simulink model "ON"  (R2025b)
settings: Solver=VariableStepAuto  StartTime=0.0  StopTime=300  FixedStep=0.5  RelTol=1e-3
InitFcn:
  | mdlWks = get_param(gcs,'ModelWorkspace');
  | a = getVariable(mdlWks,'a');
  | b = getVariable(mdlWks,'b');
  | c = getVariable(mdlWks,'c');
StopFcn:
  | fTraj = findobj("Tag","asbAUVTrajectory");
  | 
  | if isempty(fTraj)
  |    fTraj = figure("Tag","asbAUVTrajectory");
  |    axes(fTraj);
  | end
  | 
  | axTraj= gca(fTraj);
  | 
  | if exist('PositionData', 'var')
  |    plot3(axTraj,PositionData(1,1),PositionData(1,2),PositionData(1,3),'r*')
  |    hold on
  |    plot3(axTraj,PositionData(:,1),PositionData(:,2),PositionData(:,3));
  |    plot3(axTraj,PositionData(end,1),PositionData(end,2),PositionData(end,3),'g*');
  | 
  |    axTraj.XLim = [0 15];
  |    axTraj.YLim = [-10 2];
  |    axTraj.ZLim = [-2 12];
  |    axTraj.XLabel.String = 'X (m)';
  |    axTraj.YLabel.String = 'Y (m)';
  |    axTraj.ZLabel.String = 'Z (m)';
  |    grid on
  |    hold off
  | 
  |    legend(axTraj,{'Start Point','Trajectory','End Point'});
  | end
model workspace (MAT data in the model file):
  a = 1
  b = 0
  c = 1
libraries: asbAUVlib x28, dspfdesign x6, slpidlib x6, aerolibobsolete x1, aerolibasang x1, sharedutil x1, aerolibnav x1, SignalEditorBlockLib x1
(part 3 of 3)

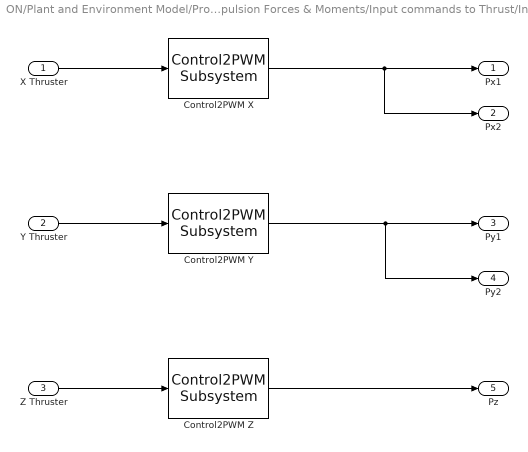
== system ON/Plant and Environment Model/Propulsion Forces & Moments/Input commands to Thrust/Input Commands to PWM ==
  X Thruster : Inport
  Y Thruster : Inport  Port=2
  Z Thruster : Inport  Port=3
  Control2PWM X : asbAUVlib/Control2PWM Subsystem  SystemSampleTime=-1  VariantActivationTime=update diagram  EmptyChoice=off  PassThrough=off  PassThroughVariantControl=(default)  EmptyChoiceVariantControl=(default)  AllowFlexibleInterface=on  Latency=0  AutoFrameSizeCalculation=off
  Control2PWM Y : asbAUVlib/Control2PWM Subsystem  SystemSampleTime=-1  VariantActivationTime=update diagram  EmptyChoice=off  PassThrough=off  PassThroughVariantControl=(default)  EmptyChoiceVariantControl=(default)  AllowFlexibleInterface=on  Latency=0  AutoFrameSizeCalculation=off
  Control2PWM Z : asbAUVlib/Control2PWM Subsystem  SystemSampleTime=-1  VariantActivationTime=update diagram  EmptyChoice=off  PassThrough=off  PassThroughVariantControl=(default)  EmptyChoiceVariantControl=(default)  AllowFlexibleInterface=on  Latency=0  AutoFrameSizeCalculation=off
  Px1 : Outport  VectorParamsAs1DForOutWhenUnconnected=off
  Px2 : Outport  Port=2  VectorParamsAs1DForOutWhenUnconnected=off
  Py1 : Outport  Port=3  VectorParamsAs1DForOutWhenUnconnected=off
  Py2 : Outport  Port=4  VectorParamsAs1DForOutWhenUnconnected=off
  Pz : Outport  Port=5  VectorParamsAs1DForOutWhenUnconnected=off
  wires:
  Control2PWM Z/1 -> Pz/1
  Y Thruster/1 -> Control2PWM Y/1
  Control2PWM Y/1 -> Py1/1, Py2/1
  Z Thruster/1 -> Control2PWM Z/1
  Control2PWM X/1 -> Px1/1, Px2/1
  X Thruster/1 -> Control2PWM X/1

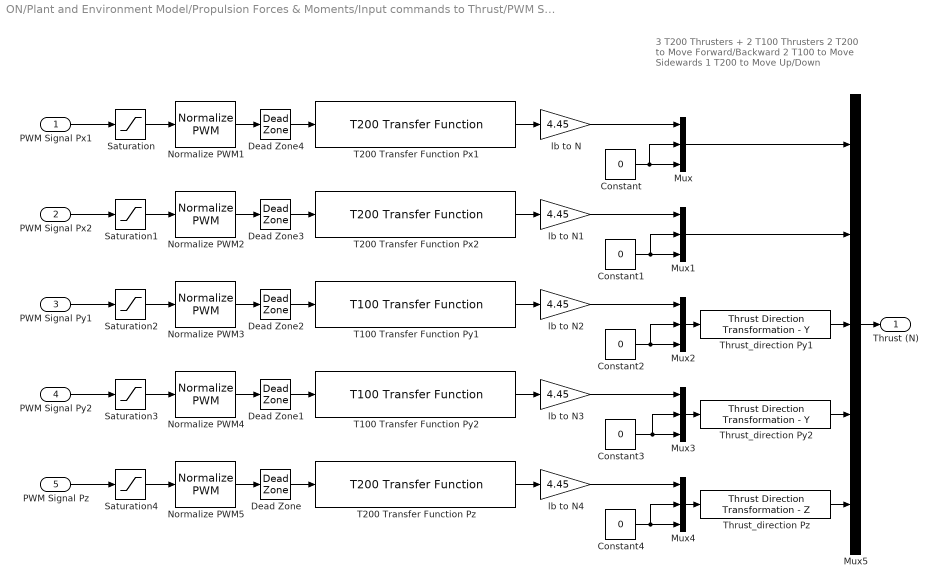
== system ON/Plant and Environment Model/Propulsion Forces & Moments/Input commands to Thrust/PWM Signals to Thrust  ==
  note: 3 T200 Thrusters + 2 T100 Thrusters
      |
      | 2 T200 to Move Forward/Backward
      | 2 T100 to Move Sidewards
      | 1 T200 to Move Up/Down
  PWM Signal Px1 : Inport
  PWM Signal Px2 : Inport  Port=2
  PWM Signal Py1 : Inport  Port=3
  PWM Signal Py2 : Inport  Port=4
  PWM Signal Pz : Inport  Port=5
  Constant{,1..4} (5 alike) : Constant  Value=0
  Dead Zone{,2..4} (4 alike) : DeadZone  LowerValue=-10  UpperValue=+10
  Dead Zone1 : DeadZone  LowerValue=-10  UpperValue=10
  Mux{,1..4} (5 alike) : Mux  Inputs=3
  Mux5 : Mux  Inputs=5
  Normalize PWM{1..5} (5 alike) : asbAUVlib/Normalize PWM  SystemSampleTime=-1  VariantActivationTime=update diagram  EmptyChoice=off  PassThrough=off  PassThroughVariantControl=(default)  EmptyChoiceVariantControl=(default)  AllowFlexibleInterface=on  Latency=0  AutoFrameSizeCalculation=off
  Saturation{,1..4} (5 alike) : Saturate  UpperLimit=1900  LowerLimit=1100
  T100 Transfer Function Py1 : asbAUVlib/T100 Transfer Function  SystemSampleTime=-1  VariantActivationTime=update diagram  EmptyChoice=off  PassThrough=off  PassThroughVariantControl=(default)  EmptyChoiceVariantControl=(default)  AllowFlexibleInterface=on  Latency=0  AutoFrameSizeCalculation=off
  T100 Transfer Function Py2 : asbAUVlib/T100 Transfer Function  SystemSampleTime=-1  VariantActivationTime=update diagram  EmptyChoice=off  PassThrough=off  PassThroughVariantControl=(default)  EmptyChoiceVariantControl=(default)  AllowFlexibleInterface=on  Latency=0  AutoFrameSizeCalculation=off
  T200 Transfer Function Px1 : asbAUVlib/T200 Transfer Function  SystemSampleTime=-1  VariantActivationTime=update diagram  EmptyChoice=off  PassThrough=off  PassThroughVariantControl=(default)  EmptyChoiceVariantControl=(default)  AllowFlexibleInterface=on  Latency=0  AutoFrameSizeCalculation=off
  T200 Transfer Function Px2 : asbAUVlib/T200 Transfer Function  SystemSampleTime=-1  VariantActivationTime=update diagram  EmptyChoice=off  PassThrough=off  PassThroughVariantControl=(default)  EmptyChoiceVariantControl=(default)  AllowFlexibleInterface=on  Latency=0  AutoFrameSizeCalculation=off
  T200 Transfer Function Pz : asbAUVlib/T200 Transfer Function  SystemSampleTime=-1  VariantActivationTime=update diagram  EmptyChoice=off  PassThrough=off  PassThroughVariantControl=(default)  EmptyChoiceVariantControl=(default)  AllowFlexibleInterface=on  Latency=0  AutoFrameSizeCalculation=off
  Thrust_direction Py1 : asbAUVlib/Thrust Direction Transformation - Y  SystemSampleTime=-1  VariantActivationTime=update diagram  EmptyChoice=off  PassThrough=off  PassThroughVariantControl=(default)  EmptyChoiceVariantControl=(default)  AllowFlexibleInterface=on  Latency=0  AutoFrameSizeCalculation=off
  Thrust_direction Py2 : asbAUVlib/Thrust Direction Transformation - Y  SystemSampleTime=-1  VariantActivationTime=update diagram  EmptyChoice=off  PassThrough=off  PassThroughVariantControl=(default)  EmptyChoiceVariantControl=(default)  AllowFlexibleInterface=on  Latency=0  AutoFrameSizeCalculation=off
  Thrust_direction Pz : asbAUVlib/Thrust Direction Transformation - Z  SystemSampleTime=-1  VariantActivationTime=update diagram  EmptyChoice=off  PassThrough=off  PassThroughVariantControl=(default)  EmptyChoiceVariantControl=(default)  AllowFlexibleInterface=on  Latency=0  AutoFrameSizeCalculation=off
  lb to N{,1..4} (5 alike) : Gain  Gain=4.45
  Thrust (N) : Outport  VectorParamsAs1DForOutWhenUnconnected=off
  wires:
  Dead Zone3/1 -> T200 Transfer Function Px2/1
  Dead Zone1/1 -> T100 Transfer Function Py2/1
  Dead Zone/1 -> T200 Transfer Function Pz/1
  Normalize PWM5/1 -> Dead Zone/1
  Normalize PWM4/1 -> Dead Zone1/1
  Normalize PWM3/1 -> Dead Zone2/1
  Normalize PWM2/1 -> Dead Zone3/1
  Saturation3/1 -> Normalize PWM4/1
  PWM Signal Py2/1 -> Saturation3/1
  Saturation4/1 -> Normalize PWM5/1
  Saturation2/1 -> Normalize PWM3/1
  Saturation1/1 -> Normalize PWM2/1
  Saturation/1 -> Normalize PWM1/1
  Normalize PWM1/1 -> Dead Zone4/1
  T100 Transfer Function Py2/1 -> lb to N3/1
  lb to N2/1 -> Mux2/1
  Mux4/1 -> Thrust_direction Pz/1
  Mux5/1 -> Thrust (N)/1
  Thrust_direction Pz/1 -> Mux5/5
  lb to N/1 -> Mux/1
  Constant1/1 -> Mux1/2, Mux1/3
  T200 Transfer Function Px2/1 -> lb to N1/1
  Mux3/1 -> Thrust_direction Py2/1
  PWM Signal Pz/1 -> Saturation4/1
  PWM Signal Px1/1 -> Saturation/1
  Constant/1 -> Mux/2, Mux/3
  Thrust_direction Py2/1 -> Mux5/4
  Thrust_direction Py1/1 -> Mux5/3
  PWM Signal Py1/1 -> Saturation2/1
  Mux1/1 -> Mux5/2
  lb to N1/1 -> Mux1/1
  lb to N4/1 -> Mux4/1
  Constant4/1 -> Mux4/3, Mux4/2
  T200 Transfer Function Pz/1 -> lb to N4/1
  Mux/1 -> Mux5/1
  Constant2/1 -> Mux2/3, Mux2/2
  Mux2/1 -> Thrust_direction Py1/1
  PWM Signal Px2/1 -> Saturation1/1
  Constant3/1 -> Mux3/2, Mux3/3
  lb to N3/1 -> Mux3/1
  Dead Zone4/1 -> T200 Transfer Function Px1/1
  T200 Transfer Function Px1/1 -> lb to N/1
  Dead Zone2/1 -> T100 Transfer Function Py1/1
  T100 Transfer Function Py1/1 -> lb to N2/1

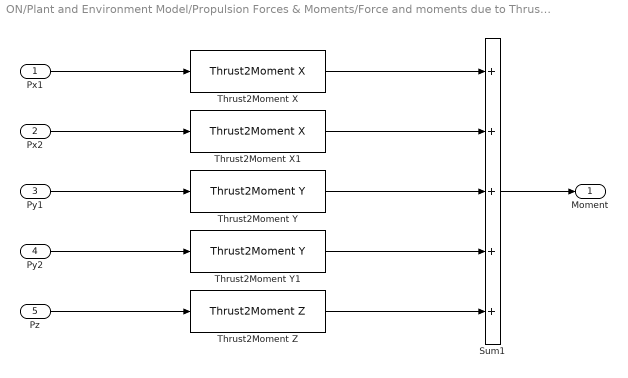
== system ON/Plant and Environment Model/Propulsion Forces & Moments/Force and moments due to Thrust/Thrust to Propulsion /Moment computation ==
  Px1 : Inport
  Px2 : Inport  Port=2
  Py1 : Inport  Port=3
  Py2 : Inport  Port=4
  Pz : Inport  Port=5
  Sum1 : Sum  Inputs=+++++
  Thrust2Moment X : asbAUVlib/Thrust2Moment X  a=0  b=-0.2  c=0
  Thrust2Moment X1 : asbAUVlib/Thrust2Moment X  a=0  b=0.2  c=0
  Thrust2Moment Y : asbAUVlib/Thrust2Moment Y  a=.2  b=0  c=0
  Thrust2Moment Y1 : asbAUVlib/Thrust2Moment Y  a=-0.2  b=0  c=0
  Thrust2Moment Z : asbAUVlib/Thrust2Moment Z  a=0  b=0  c=0
  Moment : Outport  VectorParamsAs1DForOutWhenUnconnected=off
  wires:
  Py2/1 -> Thrust2Moment Y1/1
  Px1/1 -> Thrust2Moment X/1
  Py1/1 -> Thrust2Moment Y/1
  Thrust2Moment X/1 -> Sum1/1
  Thrust2Moment X1/1 -> Sum1/2
  Thrust2Moment Z/1 -> Sum1/5
  Thrust2Moment Y1/1 -> Sum1/4
  Pz/1 -> Thrust2Moment Z/1
  Thrust2Moment Y/1 -> Sum1/3
  Sum1/1 -> Moment/1
  Px2/1 -> Thrust2Moment X1/1

== system ON/Plant and Environment Model/Propulsion Forces & Moments/Force and moments due to Thrust/Thrust to Propulsion /Thrust Transformation ==
  Thrust Inputs : Inport
  Demux1 : Demux  Outputs=5
  Thrust Px1 : Outport  VectorParamsAs1DForOutWhenUnconnected=off
  Thrust Px2 : Outport  Port=2  VectorParamsAs1DForOutWhenUnconnected=off
  Thrust Py1 : Outport  Port=3  VectorParamsAs1DForOutWhenUnconnected=off
  Thrust Py2 : Outport  Port=4  VectorParamsAs1DForOutWhenUnconnected=off
  Thrust Pz : Outport  Port=5  VectorParamsAs1DForOutWhenUnconnected=off
  wires:
  Demux1/4 -> Thrust Py2/1
  Demux1/5 -> Thrust Pz/1
  Thrust Inputs/1 -> Demux1/1
  Demux1/1 -> Thrust Px1/1
  Demux1/2 -> Thrust Px2/1
  Demux1/3 -> Thrust Py1/1
